simulink model "led_switch_control"  (R2025a)
settings: Solver=FixedStepDiscrete  StartTime=0.0  StopTime=10  FixedStep=1  RelTol=1e-3
settings Model: Creator=mahij  LastModifiedBy=mahij

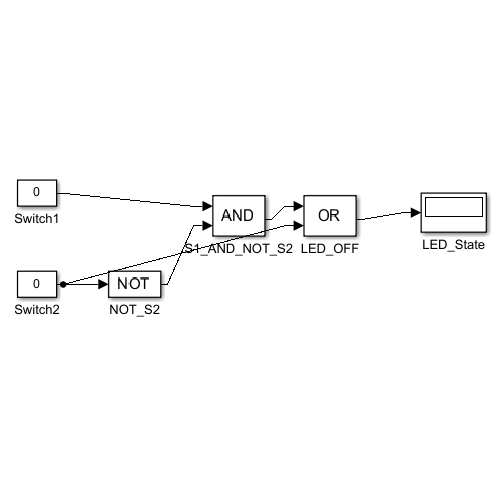
[thumbnail: Simulink's stored preview of the top-level diagram]
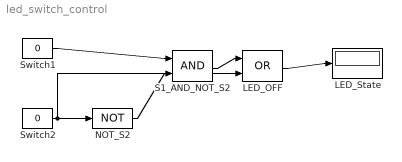
== system led_switch_control ==
  LED_OFF : Logic  Operator=OR  AllPortsSameDT=off  OutDataTypeStr=boolean
  LED_State : Display
  NOT_S2 : Logic  Operator=NOT  AllPortsSameDT=off  OutDataTypeStr=boolean
  S1_AND_NOT_S2 : Logic  AllPortsSameDT=off  OutDataTypeStr=boolean
  Switch1 : Constant  Value=0
  Switch2 : Constant  Value=0
  wires:
  Switch1/1 -> S1_AND_NOT_S2/1
  Switch2/1 -> NOT_S2/1, LED_OFF/2
  NOT_S2/1 -> S1_AND_NOT_S2/2
  S1_AND_NOT_S2/1 -> LED_OFF/1
  LED_OFF/1 -> LED_State/1
